simulink model "sens_example_sir_sim"  (R2017a)
settings: Solver=ode5  StartTime=0.0  StopTime=100  FixedStep=1  MaxStep=0.01  RelTol=1e-3  EnableMultiTasking=on
model workspace (MAT data in the model file):
  I0 = 0.1
  alpha = 0.45
  beta = 0.15
  p = [0.491750110413; 0.154394214776]
settings Model: Creator=CarlosM  LastModifiedBy=drojasd
settings DataIOCC: SaveFormat=Array  SignalLogging=off  DSMLogging=off  ReturnWorkspaceOutputs=on  OutputTimes=tout
settings OptimizationCC: LifeSpan=inf
settings DebuggingCC: UnderspecifiedInitializationDetection=Classic  MergeDetectMultiDrivingBlocksExec=none  SolverPrmCheckMsg=warning  StateNameClashWarn=warning  SFUnexpectedBacktrackingDiag=warning  SFNoUnconditionalDefaultTransitionDiag=warning  SFExecutionAtInitializationDiag=none
settings HardwareCC: ProdBitPerPointer=32  ProdBitPerSizeT=32  ProdBitPerPtrDiffT=32  ProdLargestAtomicFloat=None  ProdIntDivRoundTo=Undefined  ProdEndianess=Unspecified  ProdWordSize=32  ProdHWDeviceType=32-bit Generic
settings ModelReferenceCC: PropagateSignalLabelsOutOfModel=off
settings GRTTargetCC: TargetLangStandard=C89/C90 (ANSI)  GeneratePreprocessorConditionals=Disable all
settings ConfigComp: CovMetricSettings=dw  CovHtmlReporting=on  CovSaveCumulativeToWorkspaceVar=on  CovSaveSingleToWorkspaceVar=on  CovExternalEMLEnable=off

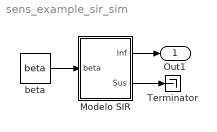
== system sens_example_sir_sim ==
  Modelo SIR : Subsystem  mask(Modelo SIR){alpha=alpha, I0=I0, S0=1-I0}
      mask prompts: alpha "Tasa de contagio (alpha)"
      mask help: Modelo Susceptibles-Infectados
  Terminator : Terminator
  beta : Constant  Value=beta
  Out1 : Outport
  wires:
  beta/1 -> Modelo SIR/1(beta)
  Modelo SIR/1(Inf) -> Out1/1
  Modelo SIR/2(Sus) -> Terminator/1

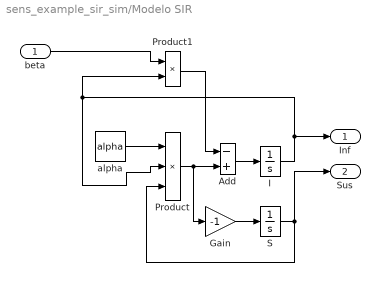
== system sens_example_sir_sim/Modelo SIR ==
  beta : Inport
  Add : Sum  Inputs=-+
  Gain : Gain  Gain=-1
  I : Integrator  InitialCondition=I0
  Product : Product  Inputs=3
  Product1 : Product
  S : Integrator  InitialCondition=S0
  alpha : Constant  Value=alpha
  Inf : Outport
  Sus : Outport  Port=2
  wires:
  Add/1 -> I/1
  I/1 -> Inf/1, Product/2, Product1/2
  Product/1 -> Add/2, Gain/1
  S/1 -> Sus/1, Product/3
  alpha/1 -> Product/1
  beta/1 -> Product1/1
  Gain/1 -> S/1
  Product1/1 -> Add/1
